simulink model "test_ffts"  (Simulink 6.2)
settings: Solver=ode45  StartTime=0.0  StopTime=300  RelTol=1e-3
undefined symbols (not defined in the file or in its folder): now
libraries: xbsIndex_r3 x1135, fft_library x1, simulink x1
(part 10 of 15)

== system test_ffts/r2_dit_fft/r2_dit_stage_2/r2_butterfly/ri_to_c ==
  re : Inport  Port=1  LatchInput=off
  im : Inport  Port=2  LatchInput=off
  concat : xbsIndex_r3/Concat  num_inputs=2  explicit_period=off  period=1  dbl_ovrd=off
  force_im : xbsIndex_r3/Reinterpret  force_arith_type=on  arith_type=Unsigned  force_bin_pt=on  bin_pt=0  force_valid=on
  force_re : xbsIndex_r3/Reinterpret  force_arith_type=on  arith_type=Unsigned  force_bin_pt=on  bin_pt=0  force_valid=on
  c : Outport
  wires:
  force_re/1 -> concat/1
  force_im/1 -> concat/2
  re/1 -> force_re/1
  concat/1 -> c/1
  im/1 -> force_im/1

== system test_ffts/r2_dit_fft/r2_dit_stage_2/r2_butterfly/ri_to_c1 ==
  re : Inport  Port=1  LatchInput=off
  im : Inport  Port=2  LatchInput=off
  concat : xbsIndex_r3/Concat  num_inputs=2  explicit_period=off  period=1  dbl_ovrd=off
  force_im : xbsIndex_r3/Reinterpret  force_arith_type=on  arith_type=Unsigned  force_bin_pt=on  bin_pt=0  force_valid=on
  force_re : xbsIndex_r3/Reinterpret  force_arith_type=on  arith_type=Unsigned  force_bin_pt=on  bin_pt=0  force_valid=on
  c : Outport
  wires:
  force_re/1 -> concat/1
  force_im/1 -> concat/2
  re/1 -> force_re/1
  concat/1 -> c/1
  im/1 -> force_im/1

== system test_ffts/r2_dit_fft/r2_dit_stage_3/biplex_commutator/delay_b ==
  in : Inport  Port=1  LatchInput=off
  slr : xbsIndex_r3/Delay  latency=8  reg_retiming=off  explicit_period=off  period=1  en=off  accept_only_valid=off  init_zero=on  dbl_ovrd=off  show_param=off
      settings: xl_area=[0, 0, 0, 0, 0, 0, 0]
  out : Outport
  wires:
  slr/1 -> out/1
  in/1 -> slr/1

== system test_ffts/r2_dit_fft/r2_dit_stage_3/biplex_commutator/delay_lo ==
  in : Inport  Port=1  LatchInput=off
  slr : xbsIndex_r3/Delay  latency=8  reg_retiming=off  explicit_period=off  period=1  en=off  accept_only_valid=off  init_zero=on  dbl_ovrd=off  show_param=off
      settings: xl_area=[0, 0, 0, 0, 0, 0, 0]
  out : Outport
  wires:
  slr/1 -> out/1
  in/1 -> slr/1

== system test_ffts/r2_dit_fft/r2_dit_stage_3/r2_butterfly/c_to_ri ==
  c : Inport  Port=1  LatchInput=off
  force_im : xbsIndex_r3/Reinterpret  force_arith_type=on  arith_type="Signed  (2's comp)"  force_bin_pt=on  bin_pt=0  force_valid=on
  force_re : xbsIndex_r3/Reinterpret  force_arith_type=on  arith_type="Signed  (2's comp)"  force_bin_pt=on  bin_pt=0  force_valid=on
  slice_im : xbsIndex_r3/Slice  mode=Lower Bit Location + Width  nbits=10  bit1=0  base1=MSB of Input  bit0=0  base0=LSB of Input  boolean_output=off  explicit_period=off  period=1  dbl_ovrd=off
  slice_re : xbsIndex_r3/Slice  mode=Upper Bit Location + Width  nbits=10  bit1=0  base1=MSB of Input  bit0=0  base0=LSB of Input  boolean_output=off  explicit_period=off  period=1  dbl_ovrd=off
  re : Outport
  im : Outport  Port=2
  wires:
  slice_re/1 -> force_re/1
  slice_im/1 -> force_im/1
  force_re/1 -> re/1
  force_im/1 -> im/1
  c/1 -> slice_re/1, slice_im/1

== system test_ffts/r2_dit_fft/r2_dit_stage_3/r2_butterfly/c_to_ri1 ==
  c : Inport  Port=1  LatchInput=off
  force_im : xbsIndex_r3/Reinterpret  force_arith_type=on  arith_type="Signed  (2's comp)"  force_bin_pt=on  bin_pt=0  force_valid=on
  force_re : xbsIndex_r3/Reinterpret  force_arith_type=on  arith_type="Signed  (2's comp)"  force_bin_pt=on  bin_pt=0  force_valid=on
  slice_im : xbsIndex_r3/Slice  mode=Lower Bit Location + Width  nbits=10  bit1=0  base1=MSB of Input  bit0=0  base0=LSB of Input  boolean_output=off  explicit_period=off  period=1  dbl_ovrd=off
  slice_re : xbsIndex_r3/Slice  mode=Upper Bit Location + Width  nbits=10  bit1=0  base1=MSB of Input  bit0=0  base0=LSB of Input  boolean_output=off  explicit_period=off  period=1  dbl_ovrd=off
  re : Outport
  im : Outport  Port=2
  wires:
  slice_re/1 -> force_re/1
  slice_im/1 -> force_im/1
  force_re/1 -> re/1
  force_im/1 -> im/1
  c/1 -> slice_re/1, slice_im/1

== system test_ffts/r2_dit_fft/r2_dit_stage_3/r2_butterfly/ri_to_c ==
  re : Inport  Port=1  LatchInput=off
  im : Inport  Port=2  LatchInput=off
  concat : xbsIndex_r3/Concat  num_inputs=2  explicit_period=off  period=1  dbl_ovrd=off
  force_im : xbsIndex_r3/Reinterpret  force_arith_type=on  arith_type=Unsigned  force_bin_pt=on  bin_pt=0  force_valid=on
  force_re : xbsIndex_r3/Reinterpret  force_arith_type=on  arith_type=Unsigned  force_bin_pt=on  bin_pt=0  force_valid=on
  c : Outport
  wires:
  force_re/1 -> concat/1
  force_im/1 -> concat/2
  re/1 -> force_re/1
  concat/1 -> c/1
  im/1 -> force_im/1

== system test_ffts/r2_dit_fft/r2_dit_stage_3/r2_butterfly/ri_to_c1 ==
  re : Inport  Port=1  LatchInput=off
  im : Inport  Port=2  LatchInput=off
  concat : xbsIndex_r3/Concat  num_inputs=2  explicit_period=off  period=1  dbl_ovrd=off
  force_im : xbsIndex_r3/Reinterpret  force_arith_type=on  arith_type=Unsigned  force_bin_pt=on  bin_pt=0  force_valid=on
  force_re : xbsIndex_r3/Reinterpret  force_arith_type=on  arith_type=Unsigned  force_bin_pt=on  bin_pt=0  force_valid=on
  c : Outport
  wires:
  force_re/1 -> concat/1
  force_im/1 -> concat/2
  re/1 -> force_re/1
  concat/1 -> c/1
  im/1 -> force_im/1

== system test_ffts/r2_dit_fft/r2_dit_stage_3/r2_twiddle/cmpy1 ==
  a_in : Inport  Port=1  LatchInput=off
  b : Inport  Port=2  LatchInput=off
  w : Inport  Port=3  LatchInput=off
  sync_in : Inport  Port=4  LatchInput=off
  Delay : xbsIndex_r3/Delay  latency=8  reg_retiming=off  explicit_period=off  period=1  en=off  accept_only_valid=off  init_zero=on  dbl_ovrd=off  show_param=off
      settings: xl_area=[1 1 0 1 0 0 0]
  Delay1 : xbsIndex_r3/Delay  latency=8  reg_retiming=off  explicit_period=off  period=1  en=off  accept_only_valid=off  init_zero=on  dbl_ovrd=off  show_param=off
      settings: xl_area=[17 34 0 34 0 0 0]
  br_add_bi : xbsIndex_r3/AddSub  mode=Addition  precision=Full  arith_type=Unsigned  n_bits=8  bin_pt=2  quantization=Truncate  overflow=Wrap  latency=1  explicit_period=off  period=1  use_carryin=off  use_carryout=off  en=off  dbl_ovrd=off  show_param=on  use_core=on  pipeline=on  use_rpm=on  gen_core=off
      settings: xl_area=[9 18 0 18 0 0 0]
  c_to_ri : Subsystem  mask(Complex to Real-Imag){n_bits=10, bin_pt=9}
      mask prompts: n_bits "Bit Width"; bin_pt "Binary Point"
      mask help: Outputs real and imaginary components of a complex input.
      settings: AttributesFormatString=10_9 r/i
      mask Help:
      | <pre>
      | Description::
      | 
      | Outputs real and imaginary components of a complex input.
      | Useful for simplifying interconnects.
      | See also: Real-Imag to Complex (ri_to_c)
      | 
      | Mask Parameters::
      | 
      | Bit Width (n_bits): Specifies the width of the real/imaginary components.
      | Assumed equal for both components.
      | 
      | Binary Point (bin_pt): Specifies the binary point location in the real/imaginary components.
      | Assumed equal for both components.
      | </pre>
  c_to_ri1 : Subsystem  mask(Complex to Real-Imag){n_bits=9, bin_pt=7}
      mask prompts: n_bits "Bit Width"; bin_pt "Binary Point"
      mask help: Outputs real and imaginary components of a complex input.
      settings: AttributesFormatString=9_7 r/i
      mask Help:
      | <pre>
      | Description::
      | 
      | Outputs real and imaginary components of a complex input.
      | Useful for simplifying interconnects.
      | See also: Real-Imag to Complex (ri_to_c)
      | 
      | Mask Parameters::
      | 
      | Bit Width (n_bits): Specifies the width of the real/imaginary components.
      | Assumed equal for both components.
      | 
      | Binary Point (bin_pt): Specifies the binary point location in the real/imaginary components.
      | Assumed equal for both components.
      | </pre>
  convert_im : xbsIndex_r3/Convert  arith_type="Signed  (2's comp)"  n_bits=10  bin_pt=9  quantization="Round  (unbiased: Even Values)"  overflow=Wrap  latency=3  explicit_period=off  period=1  dbl_ovrd=off  show_param=on  inserted_by_tool=off  pipeline=on
      settings: xl_area=[0, 0, 0, 0, 0, 0, 0]
  convert_re : xbsIndex_r3/Convert  arith_type="Signed  (2's comp)"  n_bits=10  bin_pt=9  quantization="Round  (unbiased: Even Values)"  overflow=Wrap  latency=3  explicit_period=off  period=1  dbl_ovrd=off  show_param=on  inserted_by_tool=off  pipeline=on
      settings: xl_area=[0, 0, 0, 0, 0, 0, 0]
  imim : xbsIndex_r3/Mult  precision=User Defined  arith_type="Signed  (2's comp)"  n_bits=17  bin_pt=16  quantization=Truncate  overflow=Wrap  latency=3  explicit_period=off  period=1  en=off  dbl_ovrd=off  show_param=on  mult_type=Parallel  oversample=2  use_embedded=on  pipeline=on  use_rpm=on  placement_style=Rectangular Shape  gen_core=off
      settings: xl_area=[26 52 0 26 0 1 0]
  rere : xbsIndex_r3/Mult  precision=User Defined  arith_type="Signed  (2's comp)"  n_bits=17  bin_pt=16  quantization=Truncate  overflow=Wrap  latency=3  explicit_period=off  period=1  en=off  dbl_ovrd=off  show_param=on  mult_type=Parallel  oversample=2  use_embedded=on  pipeline=on  use_rpm=on  placement_style=Rectangular Shape  gen_core=off
      settings: xl_area=[26 52 0 26 0 1 0]
  ri_to_c : Subsystem
      mask Type: Real-Imag to Complex
      mask Description: Concatenates real and imaginary inputs into a complex output.
      mask Help:
      | <pre>
      | Description::
      | 
      | Concatenates a real and imaginary input into a complex output.
      | Useful for simplifying interconnects.
      | See also: Complex to Real-Imag (c_to_ri)
      | 
      | Mask Parameters::
      | 
      | (N/A)
      | </pre>
  rr_add_ii : xbsIndex_r3/AddSub  mode=Addition  precision=User Defined  arith_type="Signed  (2's comp)"  n_bits=17  bin_pt=16  quantization=Truncate  overflow=Wrap  latency=1  explicit_period=off  period=1  use_carryin=off  use_carryout=off  en=off  dbl_ovrd=off  show_param=on  use_core=on  pipeline=on  use_rpm=on  gen_core=off
      settings: xl_area=[14 27 0 27 0 0 0]
  rr_sub_ii : xbsIndex_r3/AddSub  mode=Subtraction  precision=User Defined  arith_type="Signed  (2's comp)"  n_bits=17  bin_pt=16  quantization=Truncate  overflow=Wrap  latency=2  explicit_period=off  period=1  use_carryin=off  use_carryout=off  en=off  dbl_ovrd=off  show_param=on  use_core=on  pipeline=on  use_rpm=on  gen_core=off
      settings: xl_area=[44 44 0 69 0 0 0]
  ss_sub_rrii : xbsIndex_r3/AddSub  mode=Subtraction  precision=User Defined  arith_type="Signed  (2's comp)"  n_bits=17  bin_pt=16  quantization=Truncate  overflow=Wrap  latency=1  explicit_period=off  period=1  use_carryin=off  use_carryout=off  en=off  dbl_ovrd=off  show_param=on  use_core=on  pipeline=on  use_rpm=on  gen_core=off
      settings: xl_area=[46 29 0 90 0 0 0]
  sumsum : xbsIndex_r3/Mult  precision=User Defined  arith_type="Signed  (2's comp)"  n_bits=17  bin_pt=16  quantization=Truncate  overflow=Wrap  latency=3  explicit_period=off  period=1  en=off  dbl_ovrd=off  show_param=on  mult_type=Parallel  oversample=2  use_embedded=on  pipeline=on  use_rpm=on  placement_style=Rectangular Shape  gen_core=off
      settings: xl_area=[28 56 0 28 0 1 0]
  wr_add_wi : xbsIndex_r3/AddSub  mode=Addition  precision=Full  arith_type=Unsigned  n_bits=8  bin_pt=2  quantization=Truncate  overflow=Wrap  latency=1  explicit_period=off  period=1  use_carryin=off  use_carryout=off  en=off  dbl_ovrd=off  show_param=on  use_core=on  pipeline=on  use_rpm=on  gen_core=off
      settings: xl_area=[5 10 0 10 0 0 0]
  a_out : Outport
  bw : Outport  Port=2
  sync_out : Outport  Port=3
  wires:
  convert_im/1 -> ri_to_c/2(im)
  convert_re/1 -> ri_to_c/1(re)
  Delay1/1 -> a_out/1
  a_in/1 -> Delay1/1
  c_to_ri/2(im) -> imim/1, br_add_bi/2
  c_to_ri1/1(re) -> wr_add_wi/1, rere/2
  c_to_ri1/2(im) -> wr_add_wi/2, imim/2
  c_to_ri/1(re) -> rere/1, br_add_bi/1
  Delay/1 -> sync_out/1
  sync_in/1 -> Delay/1
  sumsum/1 -> ss_sub_rrii/1
  ri_to_c/1(c) -> bw/1
  wr_add_wi/1 -> sumsum/2
  br_add_bi/1 -> sumsum/1
  imim/1 -> rr_add_ii/1, rr_sub_ii/2
  rere/1 -> rr_sub_ii/1, rr_add_ii/2
  w/1 -> c_to_ri1/1(c)
  b/1 -> c_to_ri/1(c)
  rr_add_ii/1 -> ss_sub_rrii/2
  rr_sub_ii/1 -> convert_re/1
  ss_sub_rrii/1 -> convert_im/1

== system test_ffts/r2_dit_fft/r2_dit_stage_3/r2_twiddle/twiddle_gen1 ==
  sync_in : Inport  Port=1  LatchInput=off
  Counter : xbsIndex_r3/Counter  cnt_type=Free Running  n_bits=5  bin_pt=0  arith_type=Unsigned  start_count=0  cnt_to=Inf  cnt_by_val=1  operation=Up  explicit_period=off  period=1  load_pin=off  rst=on  en=off  dbl_ovrd=off  show_param=off  use_rpm=on  gen_core=off
      settings: xl_area=[0, 0, 0, 0, 0, 0, 0]
  addr_sel : xbsIndex_r3/Slice  mode=Upper Bit Location + Width  nbits=2  bit1=0  base1=MSB of Input  bit0=-1  base0=MSB of Input  boolean_output=off  explicit_period=off  period=1  dbl_ovrd=off
  mem_c : xbsIndex_r3/ROM  depth=4  initVector=[65536;384;47013;215973]  arith_type=Unsigned  n_bits=18  bin_pt=0  latency=1  init_zero=on  explicit_period=off  period=1  rst=off  init_reg=0  en=off  dbl_ovrd=off  show_param=on  distributed_mem=on  use_rpm=on  gen_core=off
      settings: AttributesFormatString=depth = %<depth>\ndist_mem = %<distributed_mem>  xl_area=[0, 0, 0, 0, 0, 0, 0]
  w : Outport
  wires:
  mem_c/1 -> w/1
  addr_sel/1 -> mem_c/1
  Counter/1 -> addr_sel/1
  sync_in/1 -> Counter/1

== system test_ffts/r2_dit_fft/r2_dit_stage_4/biplex_commutator/delay_b ==
  in : Inport  Port=1  LatchInput=off
  slr : xbsIndex_r3/Delay  latency=4  reg_retiming=off  explicit_period=off  period=1  en=off  accept_only_valid=off  init_zero=on  dbl_ovrd=off  show_param=off
      settings: xl_area=[0, 0, 0, 0, 0, 0, 0]
  out : Outport
  wires:
  slr/1 -> out/1
  in/1 -> slr/1

== system test_ffts/r2_dit_fft/r2_dit_stage_4/biplex_commutator/delay_lo ==
  in : Inport  Port=1  LatchInput=off
  slr : xbsIndex_r3/Delay  latency=4  reg_retiming=off  explicit_period=off  period=1  en=off  accept_only_valid=off  init_zero=on  dbl_ovrd=off  show_param=off
      settings: xl_area=[0, 0, 0, 0, 0, 0, 0]
  out : Outport
  wires:
  slr/1 -> out/1
  in/1 -> slr/1

== system test_ffts/r2_dit_fft/r2_dit_stage_4/r2_butterfly/c_to_ri ==
  c : Inport  Port=1  LatchInput=off
  force_im : xbsIndex_r3/Reinterpret  force_arith_type=on  arith_type="Signed  (2's comp)"  force_bin_pt=on  bin_pt=0  force_valid=on
  force_re : xbsIndex_r3/Reinterpret  force_arith_type=on  arith_type="Signed  (2's comp)"  force_bin_pt=on  bin_pt=0  force_valid=on
  slice_im : xbsIndex_r3/Slice  mode=Lower Bit Location + Width  nbits=11  bit1=0  base1=MSB of Input  bit0=0  base0=LSB of Input  boolean_output=off  explicit_period=off  period=1  dbl_ovrd=off
  slice_re : xbsIndex_r3/Slice  mode=Upper Bit Location + Width  nbits=11  bit1=0  base1=MSB of Input  bit0=0  base0=LSB of Input  boolean_output=off  explicit_period=off  period=1  dbl_ovrd=off
  re : Outport
  im : Outport  Port=2
  wires:
  slice_re/1 -> force_re/1
  slice_im/1 -> force_im/1
  force_re/1 -> re/1
  force_im/1 -> im/1
  c/1 -> slice_re/1, slice_im/1

== system test_ffts/r2_dit_fft/r2_dit_stage_4/r2_butterfly/c_to_ri1 ==
  c : Inport  Port=1  LatchInput=off
  force_im : xbsIndex_r3/Reinterpret  force_arith_type=on  arith_type="Signed  (2's comp)"  force_bin_pt=on  bin_pt=0  force_valid=on
  force_re : xbsIndex_r3/Reinterpret  force_arith_type=on  arith_type="Signed  (2's comp)"  force_bin_pt=on  bin_pt=0  force_valid=on
  slice_im : xbsIndex_r3/Slice  mode=Lower Bit Location + Width  nbits=11  bit1=0  base1=MSB of Input  bit0=0  base0=LSB of Input  boolean_output=off  explicit_period=off  period=1  dbl_ovrd=off
  slice_re : xbsIndex_r3/Slice  mode=Upper Bit Location + Width  nbits=11  bit1=0  base1=MSB of Input  bit0=0  base0=LSB of Input  boolean_output=off  explicit_period=off  period=1  dbl_ovrd=off
  re : Outport
  im : Outport  Port=2
  wires:
  slice_re/1 -> force_re/1
  slice_im/1 -> force_im/1
  force_re/1 -> re/1
  force_im/1 -> im/1
  c/1 -> slice_re/1, slice_im/1

== system test_ffts/r2_dit_fft/r2_dit_stage_4/r2_butterfly/ri_to_c ==
  re : Inport  Port=1  LatchInput=off
  im : Inport  Port=2  LatchInput=off
  concat : xbsIndex_r3/Concat  num_inputs=2  explicit_period=off  period=1  dbl_ovrd=off
  force_im : xbsIndex_r3/Reinterpret  force_arith_type=on  arith_type=Unsigned  force_bin_pt=on  bin_pt=0  force_valid=on
  force_re : xbsIndex_r3/Reinterpret  force_arith_type=on  arith_type=Unsigned  force_bin_pt=on  bin_pt=0  force_valid=on
  c : Outport
  wires:
  force_re/1 -> concat/1
  force_im/1 -> concat/2
  re/1 -> force_re/1
  concat/1 -> c/1
  im/1 -> force_im/1

== system test_ffts/r2_dit_fft/r2_dit_stage_4/r2_butterfly/ri_to_c1 ==
  re : Inport  Port=1  LatchInput=off
  im : Inport  Port=2  LatchInput=off
  concat : xbsIndex_r3/Concat  num_inputs=2  explicit_period=off  period=1  dbl_ovrd=off
  force_im : xbsIndex_r3/Reinterpret  force_arith_type=on  arith_type=Unsigned  force_bin_pt=on  bin_pt=0  force_valid=on
  force_re : xbsIndex_r3/Reinterpret  force_arith_type=on  arith_type=Unsigned  force_bin_pt=on  bin_pt=0  force_valid=on
  c : Outport
  wires:
  force_re/1 -> concat/1
  force_im/1 -> concat/2
  re/1 -> force_re/1
  concat/1 -> c/1
  im/1 -> force_im/1

== system test_ffts/r2_dit_fft/r2_dit_stage_4/r2_twiddle/cmpy1 ==
  a_in : Inport  Port=1  LatchInput=off
  b : Inport  Port=2  LatchInput=off
  w : Inport  Port=3  LatchInput=off
  sync_in : Inport  Port=4  LatchInput=off
  Delay : xbsIndex_r3/Delay  latency=8  reg_retiming=off  explicit_period=off  period=1  en=off  accept_only_valid=off  init_zero=on  dbl_ovrd=off  show_param=off
      settings: xl_area=[1 1 0 1 0 0 0]
  Delay1 : xbsIndex_r3/Delay  latency=8  reg_retiming=off  explicit_period=off  period=1  en=off  accept_only_valid=off  init_zero=on  dbl_ovrd=off  show_param=off
      settings: xl_area=[17 34 0 34 0 0 0]
  br_add_bi : xbsIndex_r3/AddSub  mode=Addition  precision=Full  arith_type=Unsigned  n_bits=8  bin_pt=2  quantization=Truncate  overflow=Wrap  latency=1  explicit_period=off  period=1  use_carryin=off  use_carryout=off  en=off  dbl_ovrd=off  show_param=on  use_core=on  pipeline=on  use_rpm=on  gen_core=off
      settings: xl_area=[9 18 0 18 0 0 0]
  c_to_ri : Subsystem  mask(Complex to Real-Imag){n_bits=11, bin_pt=10}
      mask prompts: n_bits "Bit Width"; bin_pt "Binary Point"
      mask help: Outputs real and imaginary components of a complex input.
      settings: AttributesFormatString=11_10 r/i
      mask Help:
      | <pre>
      | Description::
      | 
      | Outputs real and imaginary components of a complex input.
      | Useful for simplifying interconnects.
      | See also: Real-Imag to Complex (ri_to_c)
      | 
      | Mask Parameters::
      | 
      | Bit Width (n_bits): Specifies the width of the real/imaginary components.
      | Assumed equal for both components.
      | 
      | Binary Point (bin_pt): Specifies the binary point location in the real/imaginary components.
      | Assumed equal for both components.
      | </pre>
  c_to_ri1 : Subsystem  mask(Complex to Real-Imag){n_bits=9, bin_pt=7}
      mask prompts: n_bits "Bit Width"; bin_pt "Binary Point"
      mask help: Outputs real and imaginary components of a complex input.
      settings: AttributesFormatString=9_7 r/i
      mask Help:
      | <pre>
      | Description::
      | 
      | Outputs real and imaginary components of a complex input.
      | Useful for simplifying interconnects.
      | See also: Real-Imag to Complex (ri_to_c)
      | 
      | Mask Parameters::
      | 
      | Bit Width (n_bits): Specifies the width of the real/imaginary components.
      | Assumed equal for both components.
      | 
      | Binary Point (bin_pt): Specifies the binary point location in the real/imaginary components.
      | Assumed equal for both components.
      | </pre>
  convert_im : xbsIndex_r3/Convert  arith_type="Signed  (2's comp)"  n_bits=11  bin_pt=10  quantization="Round  (unbiased: Even Values)"  overflow=Wrap  latency=3  explicit_period=off  period=1  dbl_ovrd=off  show_param=on  inserted_by_tool=off  pipeline=on
      settings: xl_area=[0, 0, 0, 0, 0, 0, 0]
  convert_re : xbsIndex_r3/Convert  arith_type="Signed  (2's comp)"  n_bits=11  bin_pt=10  quantization="Round  (unbiased: Even Values)"  overflow=Wrap  latency=3  explicit_period=off  period=1  dbl_ovrd=off  show_param=on  inserted_by_tool=off  pipeline=on
      settings: xl_area=[0, 0, 0, 0, 0, 0, 0]
  imim : xbsIndex_r3/Mult  precision=User Defined  arith_type="Signed  (2's comp)"  n_bits=18  bin_pt=17  quantization=Truncate  overflow=Wrap  latency=3  explicit_period=off  period=1  en=off  dbl_ovrd=off  show_param=on  mult_type=Parallel  oversample=2  use_embedded=on  pipeline=on  use_rpm=on  placement_style=Rectangular Shape  gen_core=off
      settings: xl_area=[26 52 0 26 0 1 0]
  rere : xbsIndex_r3/Mult  precision=User Defined  arith_type="Signed  (2's comp)"  n_bits=18  bin_pt=17  quantization=Truncate  overflow=Wrap  latency=3  explicit_period=off  period=1  en=off  dbl_ovrd=off  show_param=on  mult_type=Parallel  oversample=2  use_embedded=on  pipeline=on  use_rpm=on  placement_style=Rectangular Shape  gen_core=off
      settings: xl_area=[26 52 0 26 0 1 0]
  ri_to_c : Subsystem
      mask Type: Real-Imag to Complex
      mask Description: Concatenates real and imaginary inputs into a complex output.
      mask Help:
      | <pre>
      | Description::
      | 
      | Concatenates a real and imaginary input into a complex output.
      | Useful for simplifying interconnects.
      | See also: Complex to Real-Imag (c_to_ri)
      | 
      | Mask Parameters::
      | 
      | (N/A)
      | </pre>
  rr_add_ii : xbsIndex_r3/AddSub  mode=Addition  precision=User Defined  arith_type="Signed  (2's comp)"  n_bits=18  bin_pt=17  quantization=Truncate  overflow=Wrap  latency=1  explicit_period=off  period=1  use_carryin=off  use_carryout=off  en=off  dbl_ovrd=off  show_param=on  use_core=on  pipeline=on  use_rpm=on  gen_core=off
      settings: xl_area=[14 27 0 27 0 0 0]
  rr_sub_ii : xbsIndex_r3/AddSub  mode=Subtraction  precision=User Defined  arith_type="Signed  (2's comp)"  n_bits=18  bin_pt=17  quantization=Truncate  overflow=Wrap  latency=2  explicit_period=off  period=1  use_carryin=off  use_carryout=off  en=off  dbl_ovrd=off  show_param=on  use_core=on  pipeline=on  use_rpm=on  gen_core=off
      settings: xl_area=[44 44 0 69 0 0 0]
  ss_sub_rrii : xbsIndex_r3/AddSub  mode=Subtraction  precision=User Defined  arith_type="Signed  (2's comp)"  n_bits=18  bin_pt=17  quantization=Truncate  overflow=Wrap  latency=1  explicit_period=off  period=1  use_carryin=off  use_carryout=off  en=off  dbl_ovrd=off  show_param=on  use_core=on  pipeline=on  use_rpm=on  gen_core=off
      settings: xl_area=[46 29 0 90 0 0 0]
  sumsum : xbsIndex_r3/Mult  precision=User Defined  arith_type="Signed  (2's comp)"  n_bits=18  bin_pt=17  quantization=Truncate  overflow=Wrap  latency=3  explicit_period=off  period=1  en=off  dbl_ovrd=off  show_param=on  mult_type=Parallel  oversample=2  use_embedded=on  pipeline=on  use_rpm=on  placement_style=Rectangular Shape  gen_core=off
      settings: xl_area=[28 56 0 28 0 1 0]
  wr_add_wi : xbsIndex_r3/AddSub  mode=Addition  precision=Full  arith_type=Unsigned  n_bits=8  bin_pt=2  quantization=Truncate  overflow=Wrap  latency=1  explicit_period=off  period=1  use_carryin=off  use_carryout=off  en=off  dbl_ovrd=off  show_param=on  use_core=on  pipeline=on  use_rpm=on  gen_core=off
      settings: xl_area=[5 10 0 10 0 0 0]
  a_out : Outport
  bw : Outport  Port=2
  sync_out : Outport  Port=3
  wires:
  convert_im/1 -> ri_to_c/2(im)
  convert_re/1 -> ri_to_c/1(re)
  Delay1/1 -> a_out/1
  a_in/1 -> Delay1/1
  c_to_ri/2(im) -> imim/1, br_add_bi/2
  c_to_ri1/1(re) -> wr_add_wi/1, rere/2
  c_to_ri1/2(im) -> wr_add_wi/2, imim/2
  c_to_ri/1(re) -> rere/1, br_add_bi/1
  Delay/1 -> sync_out/1
  sync_in/1 -> Delay/1
  sumsum/1 -> ss_sub_rrii/1
  ri_to_c/1(c) -> bw/1
  wr_add_wi/1 -> sumsum/2
  br_add_bi/1 -> sumsum/1
  imim/1 -> rr_add_ii/1, rr_sub_ii/2
  rere/1 -> rr_sub_ii/1, rr_add_ii/2
  w/1 -> c_to_ri1/1(c)
  b/1 -> c_to_ri/1(c)
  rr_add_ii/1 -> ss_sub_rrii/2
  rr_sub_ii/1 -> convert_re/1
  ss_sub_rrii/1 -> convert_im/1

== system test_ffts/r2_dit_fft/r2_dit_stage_4/r2_twiddle/twiddle_gen1 ==
  sync_in : Inport  Port=1  LatchInput=off
  Counter : xbsIndex_r3/Counter  cnt_type=Free Running  n_bits=5  bin_pt=0  arith_type=Unsigned  start_count=0  cnt_to=Inf  cnt_by_val=1  operation=Up  explicit_period=off  period=1  load_pin=off  rst=on  en=off  dbl_ovrd=off  show_param=off  use_rpm=on  gen_core=off
      settings: xl_area=[0, 0, 0, 0, 0, 0, 0]
  addr_sel : xbsIndex_r3/Slice  mode=Upper Bit Location + Width  nbits=3  bit1=0  base1=MSB of Input  bit0=-1  base0=MSB of Input  boolean_output=off  explicit_period=off  period=1  dbl_ovrd=off
  mem_c : xbsIndex_r3/ROM  depth=8  initVector=[65536;384;47013;215973;60879;237450;25482;202191]  arith_type=Unsigned  n_bits=18  bin_pt=0  latency=1  init_zero=on  explicit_period=off  period=1  rst=off  init_reg=0  en=off  dbl_ovrd=off  show_param=on  distributed_mem=on  use_rpm=on  gen_core=off
      settings: AttributesFormatString=depth = %<depth>\ndist_mem = %<distributed_mem>  xl_area=[0, 0, 0, 0, 0, 0, 0]
  w : Outport
  wires:
  mem_c/1 -> w/1
  addr_sel/1 -> mem_c/1
  Counter/1 -> addr_sel/1
  sync_in/1 -> Counter/1

== system test_ffts/r2_dit_fft/r2_dit_stage_5/biplex_commutator/delay_b ==
  in : Inport  Port=1  LatchInput=off
  slr : xbsIndex_r3/Delay  latency=2  reg_retiming=off  explicit_period=off  period=1  en=off  accept_only_valid=off  init_zero=on  dbl_ovrd=off  show_param=off
      settings: xl_area=[0, 0, 0, 0, 0, 0, 0]
  out : Outport
  wires:
  slr/1 -> out/1
  in/1 -> slr/1

== system test_ffts/r2_dit_fft/r2_dit_stage_5/biplex_commutator/delay_lo ==
  in : Inport  Port=1  LatchInput=off
  slr : xbsIndex_r3/Delay  latency=2  reg_retiming=off  explicit_period=off  period=1  en=off  accept_only_valid=off  init_zero=on  dbl_ovrd=off  show_param=off
      settings: xl_area=[0, 0, 0, 0, 0, 0, 0]
  out : Outport
  wires:
  slr/1 -> out/1
  in/1 -> slr/1

== system test_ffts/r2_dit_fft/r2_dit_stage_5/r2_butterfly/c_to_ri ==
  c : Inport  Port=1  LatchInput=off
  force_im : xbsIndex_r3/Reinterpret  force_arith_type=on  arith_type="Signed  (2's comp)"  force_bin_pt=on  bin_pt=0  force_valid=on
  force_re : xbsIndex_r3/Reinterpret  force_arith_type=on  arith_type="Signed  (2's comp)"  force_bin_pt=on  bin_pt=0  force_valid=on
  slice_im : xbsIndex_r3/Slice  mode=Lower Bit Location + Width  nbits=12  bit1=0  base1=MSB of Input  bit0=0  base0=LSB of Input  boolean_output=off  explicit_period=off  period=1  dbl_ovrd=off
  slice_re : xbsIndex_r3/Slice  mode=Upper Bit Location + Width  nbits=12  bit1=0  base1=MSB of Input  bit0=0  base0=LSB of Input  boolean_output=off  explicit_period=off  period=1  dbl_ovrd=off
  re : Outport
  im : Outport  Port=2
  wires:
  slice_re/1 -> force_re/1
  slice_im/1 -> force_im/1
  force_re/1 -> re/1
  force_im/1 -> im/1
  c/1 -> slice_re/1, slice_im/1

== system test_ffts/r2_dit_fft/r2_dit_stage_5/r2_butterfly/c_to_ri1 ==
  c : Inport  Port=1  LatchInput=off
  force_im : xbsIndex_r3/Reinterpret  force_arith_type=on  arith_type="Signed  (2's comp)"  force_bin_pt=on  bin_pt=0  force_valid=on
  force_re : xbsIndex_r3/Reinterpret  force_arith_type=on  arith_type="Signed  (2's comp)"  force_bin_pt=on  bin_pt=0  force_valid=on
  slice_im : xbsIndex_r3/Slice  mode=Lower Bit Location + Width  nbits=12  bit1=0  base1=MSB of Input  bit0=0  base0=LSB of Input  boolean_output=off  explicit_period=off  period=1  dbl_ovrd=off
  slice_re : xbsIndex_r3/Slice  mode=Upper Bit Location + Width  nbits=12  bit1=0  base1=MSB of Input  bit0=0  base0=LSB of Input  boolean_output=off  explicit_period=off  period=1  dbl_ovrd=off
  re : Outport
  im : Outport  Port=2
  wires:
  slice_re/1 -> force_re/1
  slice_im/1 -> force_im/1
  force_re/1 -> re/1
  force_im/1 -> im/1
  c/1 -> slice_re/1, slice_im/1

== system test_ffts/r2_dit_fft/r2_dit_stage_5/r2_butterfly/ri_to_c ==
  re : Inport  Port=1  LatchInput=off
  im : Inport  Port=2  LatchInput=off
  concat : xbsIndex_r3/Concat  num_inputs=2  explicit_period=off  period=1  dbl_ovrd=off
  force_im : xbsIndex_r3/Reinterpret  force_arith_type=on  arith_type=Unsigned  force_bin_pt=on  bin_pt=0  force_valid=on
  force_re : xbsIndex_r3/Reinterpret  force_arith_type=on  arith_type=Unsigned  force_bin_pt=on  bin_pt=0  force_valid=on
  c : Outport
  wires:
  force_re/1 -> concat/1
  force_im/1 -> concat/2
  re/1 -> force_re/1
  concat/1 -> c/1
  im/1 -> force_im/1

== system test_ffts/r2_dit_fft/r2_dit_stage_5/r2_butterfly/ri_to_c1 ==
  re : Inport  Port=1  LatchInput=off
  im : Inport  Port=2  LatchInput=off
  concat : xbsIndex_r3/Concat  num_inputs=2  explicit_period=off  period=1  dbl_ovrd=off
  force_im : xbsIndex_r3/Reinterpret  force_arith_type=on  arith_type=Unsigned  force_bin_pt=on  bin_pt=0  force_valid=on
  force_re : xbsIndex_r3/Reinterpret  force_arith_type=on  arith_type=Unsigned  force_bin_pt=on  bin_pt=0  force_valid=on
  c : Outport
  wires:
  force_re/1 -> concat/1
  force_im/1 -> concat/2
  re/1 -> force_re/1
  concat/1 -> c/1
  im/1 -> force_im/1

== system test_ffts/r2_dit_fft/r2_dit_stage_5/r2_twiddle/cmpy1 ==
  a_in : Inport  Port=1  LatchInput=off
  b : Inport  Port=2  LatchInput=off
  w : Inport  Port=3  LatchInput=off
  sync_in : Inport  Port=4  LatchInput=off
  Delay : xbsIndex_r3/Delay  latency=8  reg_retiming=off  explicit_period=off  period=1  en=off  accept_only_valid=off  init_zero=on  dbl_ovrd=off  show_param=off
      settings: xl_area=[1 1 0 1 0 0 0]
  Delay1 : xbsIndex_r3/Delay  latency=8  reg_retiming=off  explicit_period=off  period=1  en=off  accept_only_valid=off  init_zero=on  dbl_ovrd=off  show_param=off
      settings: xl_area=[17 34 0 34 0 0 0]
  br_add_bi : xbsIndex_r3/AddSub  mode=Addition  precision=Full  arith_type=Unsigned  n_bits=8  bin_pt=2  quantization=Truncate  overflow=Wrap  latency=1  explicit_period=off  period=1  use_carryin=off  use_carryout=off  en=off  dbl_ovrd=off  show_param=on  use_core=on  pipeline=on  use_rpm=on  gen_core=off
      settings: xl_area=[9 18 0 18 0 0 0]
  c_to_ri : Subsystem  mask(Complex to Real-Imag){n_bits=12, bin_pt=11}
      mask prompts: n_bits "Bit Width"; bin_pt "Binary Point"
      mask help: Outputs real and imaginary components of a complex input.
      settings: AttributesFormatString=12_11 r/i
      mask Help:
      | <pre>
      | Description::
      | 
      | Outputs real and imaginary components of a complex input.
      | Useful for simplifying interconnects.
      | See also: Real-Imag to Complex (ri_to_c)
      | 
      | Mask Parameters::
      | 
      | Bit Width (n_bits): Specifies the width of the real/imaginary components.
      | Assumed equal for both components.
      | 
      | Binary Point (bin_pt): Specifies the binary point location in the real/imaginary components.
      | Assumed equal for both components.
      | </pre>
  c_to_ri1 : Subsystem  mask(Complex to Real-Imag){n_bits=9, bin_pt=7}
      mask prompts: n_bits "Bit Width"; bin_pt "Binary Point"
      mask help: Outputs real and imaginary components of a complex input.
      settings: AttributesFormatString=9_7 r/i
      mask Help:
      | <pre>
      | Description::
      | 
      | Outputs real and imaginary components of a complex input.
      | Useful for simplifying interconnects.
      | See also: Real-Imag to Complex (ri_to_c)
      | 
      | Mask Parameters::
      | 
      | Bit Width (n_bits): Specifies the width of the real/imaginary components.
      | Assumed equal for both components.
      | 
      | Binary Point (bin_pt): Specifies the binary point location in the real/imaginary components.
      | Assumed equal for both components.
      | </pre>
  convert_im : xbsIndex_r3/Convert  arith_type="Signed  (2's comp)"  n_bits=12  bin_pt=11  quantization="Round  (unbiased: Even Values)"  overflow=Wrap  latency=3  explicit_period=off  period=1  dbl_ovrd=off  show_param=on  inserted_by_tool=off  pipeline=on
      settings: xl_area=[0, 0, 0, 0, 0, 0, 0]
  convert_re : xbsIndex_r3/Convert  arith_type="Signed  (2's comp)"  n_bits=12  bin_pt=11  quantization="Round  (unbiased: Even Values)"  overflow=Wrap  latency=3  explicit_period=off  period=1  dbl_ovrd=off  show_param=on  inserted_by_tool=off  pipeline=on
      settings: xl_area=[0, 0, 0, 0, 0, 0, 0]
  imim : xbsIndex_r3/Mult  precision=User Defined  arith_type="Signed  (2's comp)"  n_bits=19  bin_pt=18  quantization=Truncate  overflow=Wrap  latency=3  explicit_period=off  period=1  en=off  dbl_ovrd=off  show_param=on  mult_type=Parallel  oversample=2  use_embedded=on  pipeline=on  use_rpm=on  placement_style=Rectangular Shape  gen_core=off
      settings: xl_area=[26 52 0 26 0 1 0]
  rere : xbsIndex_r3/Mult  precision=User Defined  arith_type="Signed  (2's comp)"  n_bits=19  bin_pt=18  quantization=Truncate  overflow=Wrap  latency=3  explicit_period=off  period=1  en=off  dbl_ovrd=off  show_param=on  mult_type=Parallel  oversample=2  use_embedded=on  pipeline=on  use_rpm=on  placement_style=Rectangular Shape  gen_core=off
      settings: xl_area=[26 52 0 26 0 1 0]
  ri_to_c : Subsystem
      mask Type: Real-Imag to Complex
      mask Description: Concatenates real and imaginary inputs into a complex output.
      mask Help:
      | <pre>
      | Description::
      | 
      | Concatenates a real and imaginary input into a complex output.
      | Useful for simplifying interconnects.
      | See also: Complex to Real-Imag (c_to_ri)
      | 
      | Mask Parameters::
      | 
      | (N/A)
      | </pre>
  rr_add_ii : xbsIndex_r3/AddSub  mode=Addition  precision=User Defined  arith_type="Signed  (2's comp)"  n_bits=19  bin_pt=18  quantization=Truncate  overflow=Wrap  latency=1  explicit_period=off  period=1  use_carryin=off  use_carryout=off  en=off  dbl_ovrd=off  show_param=on  use_core=on  pipeline=on  use_rpm=on  gen_core=off
      settings: xl_area=[14 27 0 27 0 0 0]
  rr_sub_ii : xbsIndex_r3/AddSub  mode=Subtraction  precision=User Defined  arith_type="Signed  (2's comp)"  n_bits=19  bin_pt=18  quantization=Truncate  overflow=Wrap  latency=2  explicit_period=off  period=1  use_carryin=off  use_carryout=off  en=off  dbl_ovrd=off  show_param=on  use_core=on  pipeline=on  use_rpm=on  gen_core=off
      settings: xl_area=[44 44 0 69 0 0 0]
  ss_sub_rrii : xbsIndex_r3/AddSub  mode=Subtraction  precision=User Defined  arith_type="Signed  (2's comp)"  n_bits=19  bin_pt=18  quantization=Truncate  overflow=Wrap  latency=1  explicit_period=off  period=1  use_carryin=off  use_carryout=off  en=off  dbl_ovrd=off  show_param=on  use_core=on  pipeline=on  use_rpm=on  gen_core=off
      settings: xl_area=[46 29 0 90 0 0 0]
  sumsum : xbsIndex_r3/Mult  precision=User Defined  arith_type="Signed  (2's comp)"  n_bits=19  bin_pt=18  quantization=Truncate  overflow=Wrap  latency=3  explicit_period=off  period=1  en=off  dbl_ovrd=off  show_param=on  mult_type=Parallel  oversample=2  use_embedded=on  pipeline=on  use_rpm=on  placement_style=Rectangular Shape  gen_core=off
      settings: xl_area=[28 56 0 28 0 1 0]
  wr_add_wi : xbsIndex_r3/AddSub  mode=Addition  precision=Full  arith_type=Unsigned  n_bits=8  bin_pt=2  quantization=Truncate  overflow=Wrap  latency=1  explicit_period=off  period=1  use_carryin=off  use_carryout=off  en=off  dbl_ovrd=off  show_param=on  use_core=on  pipeline=on  use_rpm=on  gen_core=off
      settings: xl_area=[5 10 0 10 0 0 0]
  a_out : Outport
  bw : Outport  Port=2
  sync_out : Outport  Port=3
  wires:
  convert_im/1 -> ri_to_c/2(im)
  convert_re/1 -> ri_to_c/1(re)
  Delay1/1 -> a_out/1
  a_in/1 -> Delay1/1
  c_to_ri/2(im) -> imim/1, br_add_bi/2
  c_to_ri1/1(re) -> wr_add_wi/1, rere/2
  c_to_ri1/2(im) -> wr_add_wi/2, imim/2
  c_to_ri/1(re) -> rere/1, br_add_bi/1
  Delay/1 -> sync_out/1
  sync_in/1 -> Delay/1
  sumsum/1 -> ss_sub_rrii/1
  ri_to_c/1(c) -> bw/1
  wr_add_wi/1 -> sumsum/2
  br_add_bi/1 -> sumsum/1
  imim/1 -> rr_add_ii/1, rr_sub_ii/2
  rere/1 -> rr_sub_ii/1, rr_add_ii/2
  w/1 -> c_to_ri1/1(c)
  b/1 -> c_to_ri/1(c)
  rr_add_ii/1 -> ss_sub_rrii/2
  rr_sub_ii/1 -> convert_re/1
  ss_sub_rrii/1 -> convert_im/1

== system test_ffts/r2_dit_fft/r2_dit_stage_5/r2_twiddle/twiddle_gen1 ==
  sync_in : Inport  Port=1  LatchInput=off
  Counter : xbsIndex_r3/Counter  cnt_type=Free Running  n_bits=5  bin_pt=0  arith_type=Unsigned  start_count=0  cnt_to=Inf  cnt_by_val=1  operation=Up  explicit_period=off  period=1  load_pin=off  rst=on  en=off  dbl_ovrd=off  show_param=off  use_rpm=on  gen_core=off
      settings: xl_area=[0, 0, 0, 0, 0, 0, 0]
  addr_sel : xbsIndex_r3/Slice  mode=Upper Bit Location + Width  nbits=4  bit1=0  base1=MSB of Input  bit0=-1  base0=MSB of Input  boolean_output=off  explicit_period=off  period=1  dbl_ovrd=off
  mem_c : xbsIndex_r3/ROM  depth=16  initVector=[65536;384;47013;215973;60879;237450;25482;202191;64999;249730;36758;208313;54713;226198;13186;198119]  arith_type=Unsigned  n_bits=18  bin_pt=0  latency=1  init_zero=on  explicit_period=off  period=1  rst=off  init_reg=0  en=off  dbl_ovrd=off  show_param=on  distributed_mem=on  use_rpm=on  gen_core=off
      settings: AttributesFormatString=depth = %<depth>\ndist_mem = %<distributed_mem>  xl_area=[0, 0, 0, 0, 0, 0, 0]
  w : Outport
  wires:
  mem_c/1 -> w/1
  addr_sel/1 -> mem_c/1
  Counter/1 -> addr_sel/1
  sync_in/1 -> Counter/1

== system test_ffts/r2_dit_fft/r2_dit_stage_6/biplex_commutator/delay_b ==
  in : Inport  Port=1  LatchInput=off
  slr : xbsIndex_r3/Delay  latency=1  reg_retiming=off  explicit_period=off  period=1  en=off  accept_only_valid=off  init_zero=on  dbl_ovrd=off  show_param=off
      settings: xl_area=[0, 0, 0, 0, 0, 0, 0]
  out : Outport
  wires:
  slr/1 -> out/1
  in/1 -> slr/1

== system test_ffts/r2_dit_fft/r2_dit_stage_6/biplex_commutator/delay_lo ==
  in : Inport  Port=1  LatchInput=off
  slr : xbsIndex_r3/Delay  latency=1  reg_retiming=off  explicit_period=off  period=1  en=off  accept_only_valid=off  init_zero=on  dbl_ovrd=off  show_param=off
      settings: xl_area=[0, 0, 0, 0, 0, 0, 0]
  out : Outport
  wires:
  slr/1 -> out/1
  in/1 -> slr/1

== system test_ffts/r2_dit_fft/r2_dit_stage_6/r2_butterfly/c_to_ri ==
  c : Inport  Port=1  LatchInput=off
  force_im : xbsIndex_r3/Reinterpret  force_arith_type=on  arith_type="Signed  (2's comp)"  force_bin_pt=on  bin_pt=0  force_valid=on
  force_re : xbsIndex_r3/Reinterpret  force_arith_type=on  arith_type="Signed  (2's comp)"  force_bin_pt=on  bin_pt=0  force_valid=on
  slice_im : xbsIndex_r3/Slice  mode=Lower Bit Location + Width  nbits=13  bit1=0  base1=MSB of Input  bit0=0  base0=LSB of Input  boolean_output=off  explicit_period=off  period=1  dbl_ovrd=off
  slice_re : xbsIndex_r3/Slice  mode=Upper Bit Location + Width  nbits=13  bit1=0  base1=MSB of Input  bit0=0  base0=LSB of Input  boolean_output=off  explicit_period=off  period=1  dbl_ovrd=off
  re : Outport
  im : Outport  Port=2
  wires:
  slice_re/1 -> force_re/1
  slice_im/1 -> force_im/1
  force_re/1 -> re/1
  force_im/1 -> im/1
  c/1 -> slice_re/1, slice_im/1

== system test_ffts/r2_dit_fft/r2_dit_stage_6/r2_butterfly/c_to_ri1 ==
  c : Inport  Port=1  LatchInput=off
  force_im : xbsIndex_r3/Reinterpret  force_arith_type=on  arith_type="Signed  (2's comp)"  force_bin_pt=on  bin_pt=0  force_valid=on
  force_re : xbsIndex_r3/Reinterpret  force_arith_type=on  arith_type="Signed  (2's comp)"  force_bin_pt=on  bin_pt=0  force_valid=on
  slice_im : xbsIndex_r3/Slice  mode=Lower Bit Location + Width  nbits=13  bit1=0  base1=MSB of Input  bit0=0  base0=LSB of Input  boolean_output=off  explicit_period=off  period=1  dbl_ovrd=off
  slice_re : xbsIndex_r3/Slice  mode=Upper Bit Location + Width  nbits=13  bit1=0  base1=MSB of Input  bit0=0  base0=LSB of Input  boolean_output=off  explicit_period=off  period=1  dbl_ovrd=off
  re : Outport
  im : Outport  Port=2
  wires:
  slice_re/1 -> force_re/1
  slice_im/1 -> force_im/1
  force_re/1 -> re/1
  force_im/1 -> im/1
  c/1 -> slice_re/1, slice_im/1

== system test_ffts/r2_dit_fft/r2_dit_stage_6/r2_butterfly/ri_to_c ==
  re : Inport  Port=1  LatchInput=off
  im : Inport  Port=2  LatchInput=off
  concat : xbsIndex_r3/Concat  num_inputs=2  explicit_period=off  period=1  dbl_ovrd=off
  force_im : xbsIndex_r3/Reinterpret  force_arith_type=on  arith_type=Unsigned  force_bin_pt=on  bin_pt=0  force_valid=on
  force_re : xbsIndex_r3/Reinterpret  force_arith_type=on  arith_type=Unsigned  force_bin_pt=on  bin_pt=0  force_valid=on
  c : Outport
  wires:
  force_re/1 -> concat/1
  force_im/1 -> concat/2
  re/1 -> force_re/1
  concat/1 -> c/1
  im/1 -> force_im/1

== system test_ffts/r2_dit_fft/r2_dit_stage_6/r2_butterfly/ri_to_c1 ==
  re : Inport  Port=1  LatchInput=off
  im : Inport  Port=2  LatchInput=off
  concat : xbsIndex_r3/Concat  num_inputs=2  explicit_period=off  period=1  dbl_ovrd=off
  force_im : xbsIndex_r3/Reinterpret  force_arith_type=on  arith_type=Unsigned  force_bin_pt=on  bin_pt=0  force_valid=on
  force_re : xbsIndex_r3/Reinterpret  force_arith_type=on  arith_type=Unsigned  force_bin_pt=on  bin_pt=0  force_valid=on
  c : Outport
  wires:
  force_re/1 -> concat/1
  force_im/1 -> concat/2
  re/1 -> force_re/1
  concat/1 -> c/1
  im/1 -> force_im/1

== system test_ffts/r2_dit_fft/r2_dit_stage_6/r2_twiddle/cmpy1 ==
  a_in : Inport  Port=1  LatchInput=off
  b : Inport  Port=2  LatchInput=off
  w : Inport  Port=3  LatchInput=off
  sync_in : Inport  Port=4  LatchInput=off
  Delay : xbsIndex_r3/Delay  latency=8  reg_retiming=off  explicit_period=off  period=1  en=off  accept_only_valid=off  init_zero=on  dbl_ovrd=off  show_param=off
      settings: xl_area=[1 1 0 1 0 0 0]
  Delay1 : xbsIndex_r3/Delay  latency=8  reg_retiming=off  explicit_period=off  period=1  en=off  accept_only_valid=off  init_zero=on  dbl_ovrd=off  show_param=off
      settings: xl_area=[17 34 0 34 0 0 0]
  br_add_bi : xbsIndex_r3/AddSub  mode=Addition  precision=Full  arith_type=Unsigned  n_bits=8  bin_pt=2  quantization=Truncate  overflow=Wrap  latency=1  explicit_period=off  period=1  use_carryin=off  use_carryout=off  en=off  dbl_ovrd=off  show_param=on  use_core=on  pipeline=on  use_rpm=on  gen_core=off
      settings: xl_area=[9 18 0 18 0 0 0]
  c_to_ri : Subsystem  mask(Complex to Real-Imag){n_bits=13, bin_pt=12}
      mask prompts: n_bits "Bit Width"; bin_pt "Binary Point"
      mask help: Outputs real and imaginary components of a complex input.
      settings: AttributesFormatString=13_12 r/i
      mask Help:
      | <pre>
      | Description::
      | 
      | Outputs real and imaginary components of a complex input.
      | Useful for simplifying interconnects.
      | See also: Real-Imag to Complex (ri_to_c)
      | 
      | Mask Parameters::
      | 
      | Bit Width (n_bits): Specifies the width of the real/imaginary components.
      | Assumed equal for both components.
      | 
      | Binary Point (bin_pt): Specifies the binary point location in the real/imaginary components.
      | Assumed equal for both components.
      | </pre>
  c_to_ri1 : Subsystem  mask(Complex to Real-Imag){n_bits=9, bin_pt=7}
      mask prompts: n_bits "Bit Width"; bin_pt "Binary Point"
      mask help: Outputs real and imaginary components of a complex input.
      settings: AttributesFormatString=9_7 r/i
      mask Help:
      | <pre>
      | Description::
      | 
      | Outputs real and imaginary components of a complex input.
      | Useful for simplifying interconnects.
      | See also: Real-Imag to Complex (ri_to_c)
      | 
      | Mask Parameters::
      | 
      | Bit Width (n_bits): Specifies the width of the real/imaginary components.
      | Assumed equal for both components.
      | 
      | Binary Point (bin_pt): Specifies the binary point location in the real/imaginary components.
      | Assumed equal for both components.
      | </pre>
  convert_im : xbsIndex_r3/Convert  arith_type="Signed  (2's comp)"  n_bits=13  bin_pt=12  quantization="Round  (unbiased: Even Values)"  overflow=Wrap  latency=3  explicit_period=off  period=1  dbl_ovrd=off  show_param=on  inserted_by_tool=off  pipeline=on
      settings: xl_area=[0, 0, 0, 0, 0, 0, 0]
  convert_re : xbsIndex_r3/Convert  arith_type="Signed  (2's comp)"  n_bits=13  bin_pt=12  quantization="Round  (unbiased: Even Values)"  overflow=Wrap  latency=3  explicit_period=off  period=1  dbl_ovrd=off  show_param=on  inserted_by_tool=off  pipeline=on
      settings: xl_area=[0, 0, 0, 0, 0, 0, 0]
  imim : xbsIndex_r3/Mult  precision=User Defined  arith_type="Signed  (2's comp)"  n_bits=20  bin_pt=19  quantization=Truncate  overflow=Wrap  latency=3  explicit_period=off  period=1  en=off  dbl_ovrd=off  show_param=on  mult_type=Parallel  oversample=2  use_embedded=on  pipeline=on  use_rpm=on  placement_style=Rectangular Shape  gen_core=off
      settings: xl_area=[26 52 0 26 0 1 0]
  rere : xbsIndex_r3/Mult  precision=User Defined  arith_type="Signed  (2's comp)"  n_bits=20  bin_pt=19  quantization=Truncate  overflow=Wrap  latency=3  explicit_period=off  period=1  en=off  dbl_ovrd=off  show_param=on  mult_type=Parallel  oversample=2  use_embedded=on  pipeline=on  use_rpm=on  placement_style=Rectangular Shape  gen_core=off
      settings: xl_area=[26 52 0 26 0 1 0]
  ri_to_c : Subsystem
      mask Type: Real-Imag to Complex
      mask Description: Concatenates real and imaginary inputs into a complex output.
      mask Help:
      | <pre>
      | Description::
      | 
      | Concatenates a real and imaginary input into a complex output.
      | Useful for simplifying interconnects.
      | See also: Complex to Real-Imag (c_to_ri)
      | 
      | Mask Parameters::
      | 
      | (N/A)
      | </pre>
  rr_add_ii : xbsIndex_r3/AddSub  mode=Addition  precision=User Defined  arith_type="Signed  (2's comp)"  n_bits=20  bin_pt=19  quantization=Truncate  overflow=Wrap  latency=1  explicit_period=off  period=1  use_carryin=off  use_carryout=off  en=off  dbl_ovrd=off  show_param=on  use_core=on  pipeline=on  use_rpm=on  gen_core=off
      settings: xl_area=[14 27 0 27 0 0 0]
  rr_sub_ii : xbsIndex_r3/AddSub  mode=Subtraction  precision=User Defined  arith_type="Signed  (2's comp)"  n_bits=20  bin_pt=19  quantization=Truncate  overflow=Wrap  latency=2  explicit_period=off  period=1  use_carryin=off  use_carryout=off  en=off  dbl_ovrd=off  show_param=on  use_core=on  pipeline=on  use_rpm=on  gen_core=off
      settings: xl_area=[44 44 0 69 0 0 0]
  ss_sub_rrii : xbsIndex_r3/AddSub  mode=Subtraction  precision=User Defined  arith_type="Signed  (2's comp)"  n_bits=20  bin_pt=19  quantization=Truncate  overflow=Wrap  latency=1  explicit_period=off  period=1  use_carryin=off  use_carryout=off  en=off  dbl_ovrd=off  show_param=on  use_core=on  pipeline=on  use_rpm=on  gen_core=off
      settings: xl_area=[46 29 0 90 0 0 0]
  sumsum : xbsIndex_r3/Mult  precision=User Defined  arith_type="Signed  (2's comp)"  n_bits=20  bin_pt=19  quantization=Truncate  overflow=Wrap  latency=3  explicit_period=off  period=1  en=off  dbl_ovrd=off  show_param=on  mult_type=Parallel  oversample=2  use_embedded=on  pipeline=on  use_rpm=on  placement_style=Rectangular Shape  gen_core=off
      settings: xl_area=[28 56 0 28 0 1 0]
  wr_add_wi : xbsIndex_r3/AddSub  mode=Addition  precision=Full  arith_type=Unsigned  n_bits=8  bin_pt=2  quantization=Truncate  overflow=Wrap  latency=1  explicit_period=off  period=1  use_carryin=off  use_carryout=off  en=off  dbl_ovrd=off  show_param=on  use_core=on  pipeline=on  use_rpm=on  gen_core=off
      settings: xl_area=[5 10 0 10 0 0 0]
  a_out : Outport
  bw : Outport  Port=2
  sync_out : Outport  Port=3
  wires:
  convert_im/1 -> ri_to_c/2(im)
  convert_re/1 -> ri_to_c/1(re)
  Delay1/1 -> a_out/1
  a_in/1 -> Delay1/1
  c_to_ri/2(im) -> imim/1, br_add_bi/2
  c_to_ri1/1(re) -> wr_add_wi/1, rere/2
  c_to_ri1/2(im) -> wr_add_wi/2, imim/2
  c_to_ri/1(re) -> rere/1, br_add_bi/1
  Delay/1 -> sync_out/1
  sync_in/1 -> Delay/1
  sumsum/1 -> ss_sub_rrii/1
  ri_to_c/1(c) -> bw/1
  wr_add_wi/1 -> sumsum/2
  br_add_bi/1 -> sumsum/1
  imim/1 -> rr_add_ii/1, rr_sub_ii/2
  rere/1 -> rr_sub_ii/1, rr_add_ii/2
  w/1 -> c_to_ri1/1(c)
  b/1 -> c_to_ri/1(c)
  rr_add_ii/1 -> ss_sub_rrii/2
  rr_sub_ii/1 -> convert_re/1
  ss_sub_rrii/1 -> convert_im/1

== system test_ffts/r2_dit_fft/r2_dit_stage_6/r2_twiddle/twiddle_gen1 ==
  sync_in : Inport  Port=1  LatchInput=off
  Counter : xbsIndex_r3/Counter  cnt_type=Free Running  n_bits=5  bin_pt=0  arith_type=Unsigned  start_count=0  cnt_to=Inf  cnt_by_val=1  operation=Up  explicit_period=off  period=1  load_pin=off  rst=on  en=off  dbl_ovrd=off  show_param=off  use_rpm=on  gen_core=off
      settings: xl_area=[0, 0, 0, 0, 0, 0, 0]
  addr_sel : xbsIndex_r3/Slice  mode=Upper Bit Location + Width  nbits=5  bit1=0  base1=MSB of Input  bit0=-1  base0=MSB of Input  boolean_output=off  explicit_period=off  period=1  dbl_ovrd=off
  mem_c : xbsIndex_r3/ROM  depth=32  initVector=[65536;384;47013;215973;60879;237450;25482;202191;64999;249730;36758;208313;54713;226198;13186;198119;65523;255873;41885;211887;58308;231823;19334;200155;62939;243590;31119;204740;51119;221085;7041;197619]  arith_type=Unsigned  n_bits=18  bin_pt=0  latency=1  init_zero=on  explicit_period=off  period=1  rst=off  init_reg=0  en=off  dbl_ovrd=off  show_param=on  distributed_mem=on  use_rpm=on  gen_core=off
      settings: AttributesFormatString=depth = %<depth>\ndist_mem = %<distributed_mem>  xl_area=[0, 0, 0, 0, 0, 0, 0]
  w : Outport
  wires:
  mem_c/1 -> w/1
  addr_sel/1 -> mem_c/1
  Counter/1 -> addr_sel/1
  sync_in/1 -> Counter/1
